simulink library "asbCubeSatActuatorsLib"  (R2020b)
settings: Solver=VariableStepAuto  StartTime=0.0  StopTime=10.0  RelTol=1e-3
libraries: asbCubeSatBlockLib x2
settings Model: Creator=The MathWorks, Inc.  LastModifiedBy=The MathWorks, Inc.
settings DataIOCC: ReturnWorkspaceOutputs=off
settings DebuggingCC: ArithmeticOperatorsInVariantConditions=warning

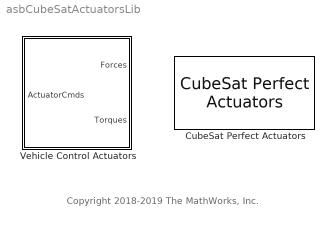
== system asbCubeSatActuatorsLib ==
  note: Copyright 2018-2019 The MathWorks, Inc.
  CubeSat Perfect Actuators : asbCubeSatBlockLib/Actuators/CubeSat Perfect Actuators  SystemSampleTime=-1
  Vehicle Control Actuators : Subsystem  RequirementInfo={} %GIDa_fba6ccff_ebba_4f2b_aabb_40150f996586

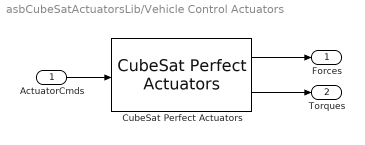
== system asbCubeSatActuatorsLib/Vehicle Control Actuators ==
  ActuatorCmds : Inport  RequirementInfo={} %GIDa_020f38c4_9e26_4002_9065_5d46819fcfcb
  CubeSat Perfect Actuators : asbCubeSatBlockLib/Actuators/CubeSat Perfect Actuators  SystemSampleTime=-1
  " Forces" : Outport  RequirementInfo={} %GIDa_e46e2c30_d205_4036_910c_a099c6c54d17  VectorParamsAs1DForOutWhenUnconnected=off
  " Torques" : Outport  RequirementInfo={} %GIDa_67b5453a_f72e_4aa8_be3c_a57a924d68da  Port=2  VectorParamsAs1DForOutWhenUnconnected=off
  wires:
  ActuatorCmds/1 -> CubeSat Perfect Actuators/1
  CubeSat Perfect Actuators/2 -> " Torques"/1
  CubeSat Perfect Actuators/1 -> " Forces"/1
